simulink model "IntroSLModel"  (R2018b)
settings: Solver=VariableStepAuto  StartTime=0.0  StopTime=50.0  MaxStep=0.05  RelTol=1e-3
undefined symbols (not defined in the file or in its folder): b, k, m
libraries: simulink x1
settings Model: Creator=carne  LastModifiedBy=carne

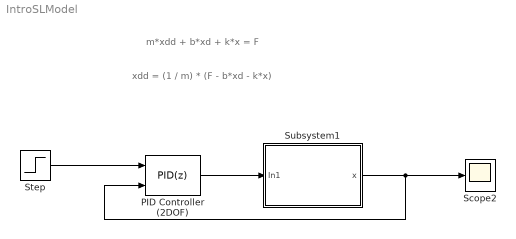
== system IntroSLModel ==
  note: xdd = (1 / m) * (F - b*xd - k*x)
  note: m*xdd + b*xd + k*x = F
  PID Controller (2DOF) : simulink/Continuous/PID Controller (2DOF)  Controller=PID  Form=Parallel  TimeDomain=Discrete-time  SampleTime=0.01  IntegratorMethod=Forward Euler  FilterMethod=Forward Euler  ControllerParametersSource=internal  P=0.612281279462149  I=0.0807782788695867  D=1.13502957342664  UseFilter=on  N=83.9593470670877  b=0.89901174780258  c=0.00667653462382807  TunerSelectOption=Transfer Function Based (PID Tuner App)  InitialConditionSource=internal  InitialConditionForIntegrator=0  InitialConditionForFilter=0  DifferentiatorICPrevScaledInput=0  ExternalReset=none  TrackingMode=off  Kt=1  LimitOutput=off  UpperSaturationLimit=inf  LowerSaturationLimit=-inf  LinearizeAsGain=on  AntiWindupMode=none  Kb=1  POutMin=[]  POutMax=[]  IOutMin=[]  IOutMax=[]  DOutMin=[]  DOutMax=[]  NOutMin=[]  NOutMax=[]  bOutMin=[]  bOutMax=[]  cOutMin=[]  cOutMax=[]  SumOutMin=[]  SumOutMax=[]  SaturationOutMin=[]  SaturationOutMax=[]  PParamMin=[]  PParamMax=[]  IParamMin=[]  IParamMax=[]  DParamMin=[]  DParamMax=[]  NParamMin=[]  NParamMax=[]  bParamMin=[]  bParamMax=[]  cParamMin=[]  cParamMax=[]  KbParamMin=[]  KbParamMax=[]  KtParamMin=[]  KtParamMax=[]  KbOutMin=[]  KbOutMax=[]  KtOutMin=[]  KtOutMax=[]  IntegratorOutMin=[]  IntegratorOutMax=[]  FilterOutMin=[]  FilterOutMax=[]  SumI1OutMin=[]  SumI1OutMax=[]  SumI2OutMin=[]  SumI2OutMax=[]  SumI3OutMin=[]  SumI3OutMax=[]  SumI4OutMin=[]  SumI4OutMax=[]  SumDOutMin=[]  SumDOutMax=[]  Sum1OutMin=[]  Sum1OutMax=[]  Sum2OutMin=[]  Sum2OutMax=[]  Sum3OutMin=[]  Sum3OutMax=[]  DifferentiatorOutMin=[]  DifferentiatorOutMax=[]  FilterDiffOutCoefMin=[]  FilterDiffOutCoefMax=[]  ReciprocalOutMin=[]  ReciprocalOutMax=[]  SumDenOutMin=[]  SumDenOutMax=[]  SumNumOutMin=[]  SumNumOutMax=[]  DivideOutMin=[]  DivideOutMax=[]  IntegratorContinuousStateAttributes=''  IntegratorStateMustResolveToSignalObject=off  IntegratorRTWStateStorageClass=Auto  FilterContinuousStateAttributes=''  FilterStateMustResolveToSignalObject=off  FilterRTWStateStorageClass=Auto  ParallelPVariant=InternalParameters  IdealPVariant=Disabled  IVariant=InternalParameters  DVariant=InternalParameters  bVariant=InternalParameters  cVariant=InternalParameters  IntegratorVariant=Discrete  SatVariant=Disabled  AWVariant=Passthrough  PCopyVariant=Disabled  TRVariant=Disabled  FdbkBlocksVariant=Forward  IdealPFdbkVariant=Disabled  SatFdbkVariant=Disabled  DerivativeFilterVariant=ForwardEulerFilter  NVariant=InternalParameters  NCopyVariant=Disabled  FilterICVariant=InternalICsFilter  IntegratorICVariant=InternalICs  ExternalResetVariant=Disabled  TRSumVariant=Passthrough  SumFdbkVariant=Disabled  SumVariant=Sum_PID
  Scope2 : Scope
  Step : Step  SampleTime=0
  Subsystem1 : Subsystem  mask{m=m, k=k / 2, b=b}
      mask prompts: m "Mass"; k "Spring"; b "Damper"
      mask Display: disp('My Subsystem')
  wires:
  Subsystem1/1(x) -> PID Controller (2DOF)/2, Scope2/1
  Step/1 -> PID Controller (2DOF)/1
  PID Controller (2DOF)/1 -> Subsystem1/1(In1)

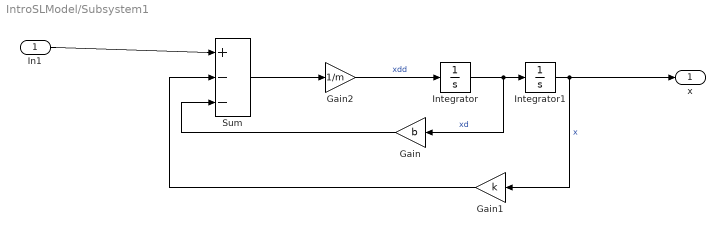
== system IntroSLModel/Subsystem1 ==
  In1 : Inport
  Gain : Gain  Gain=b
  Gain1 : Gain  Gain=k
  Gain2 : Gain  Gain=1/m
  Integrator : Integrator
  Integrator1 : Integrator
  Sum : Sum  Inputs=+|--
  x : Outport
  wires:
  Gain2/1 -> Integrator/1  "xdd"
  Sum/1 -> Gain2/1
  In1/1 -> Sum/1
  Gain1/1 -> Sum/2
  Gain/1 -> Sum/3
  Integrator1/1 -> x/1, Gain1/1  "x"
  Integrator/1 -> Gain/1, Integrator1/1  "xd"
